simulink library "GPENMPC_Demo_Connections"  (R2026a)
settings: Solver=VariableStepAuto
settings Model: Creator=Yuhao  LastModifiedBy=Yuhao

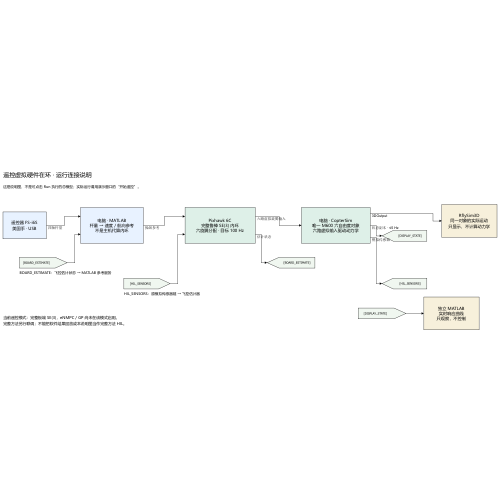
[thumbnail: Simulink's stored preview of the top-level diagram]
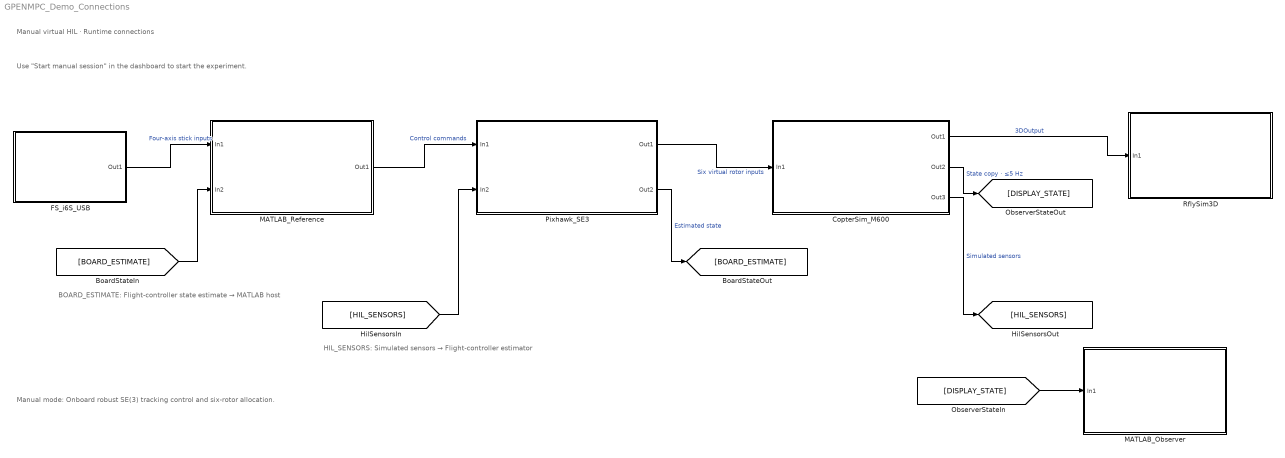
== system GPENMPC_Demo_Connections ==
  note: Manual virtual HIL · Runtime connections
  note: Use "Start manual session" in the dashboard to start the experiment.
  note: BOARD_ESTIMATE: Flight-controller state estimate → MATLAB host
  note: HIL_SENSORS: Simulated sensors → Flight-controller estimator
  note: Manual mode: Onboard robust SE(3) tracking control and six-rotor allocation.
  CopterSim_M600 : Subsystem
      mask Display: disp(sprintf('Host · CopterSim\nM600 six-degree-of-freedom dynamics\nRotor inputs and simulated sensors'))
  FS_i6S_USB : Subsystem
      mask Display: disp(sprintf('FS-i6S transmitter\nUSB stick inputs'))
  MATLAB_Observer : Subsystem
      mask Display: disp(sprintf('MATLAB live dashboard\nFlight state\nEnvironment and control response'))
  MATLAB_Reference : Subsystem
      mask Display: disp(sprintf('Host · MATLAB\nStick input processing\nVelocity and yaw-rate commands'))
  Pixhawk_SE3 : Subsystem
      mask Display: disp(sprintf('Pixhawk 6C\nReference shaping\nRobust SE(3) tracking and six-rotor allocation'))
  RflySim3D : Subsystem
      mask Display: disp(sprintf('RflySim3D\nFlight animation\nScene and motion display'))
  wires:
  FS_i6S_USB/1(Out1) -> MATLAB_Reference/1(In1)  "Four-axis stick inputs"
  MATLAB_Reference/1(Out1) -> Pixhawk_SE3/1(In1)  "Control commands"
  Pixhawk_SE3/1(Out1) -> CopterSim_M600/1(In1)  "Six virtual rotor inputs"
  Pixhawk_SE3/2(Out2) -> [BOARD_ESTIMATE]  "Estimated state"
  [BOARD_ESTIMATE] -> MATLAB_Reference/2(In2)
  CopterSim_M600/3(Out3) -> [HIL_SENSORS]  "Simulated sensors"
  [HIL_SENSORS] -> Pixhawk_SE3/2(In2)
  CopterSim_M600/2(Out2) -> [DISPLAY_STATE]  "State copy · ≤5 Hz"
  [DISPLAY_STATE] -> MATLAB_Observer/1(In1)
  CopterSim_M600/1(Out1) -> RflySim3D/1(In1)  "3DOutput"

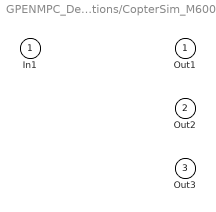
== system GPENMPC_Demo_Connections/CopterSim_M600 ==
  In1 : Inport
  Out1 : Outport
  Out2 : Outport  Port=2
  Out3 : Outport  Port=3

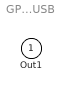
== system GPENMPC_Demo_Connections/FS_i6S_USB ==
  Out1 : Outport

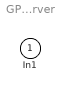
== system GPENMPC_Demo_Connections/MATLAB_Observer ==
  In1 : Inport

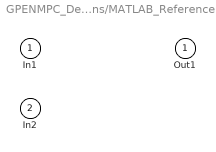
== system GPENMPC_Demo_Connections/MATLAB_Reference ==
  In1 : Inport
  In2 : Inport  Port=2
  Out1 : Outport

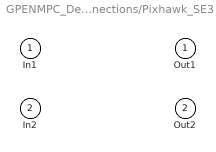
== system GPENMPC_Demo_Connections/Pixhawk_SE3 ==
  In1 : Inport
  In2 : Inport  Port=2
  Out1 : Outport
  Out2 : Outport  Port=2

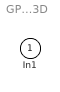
== system GPENMPC_Demo_Connections/RflySim3D ==
  In1 : Inport
